simulink model "EM_SYS_simulink"  (R2021a)
settings: Solver=VariableStepAuto  StartTime=0.0  StopTime=10.0  MaxStep=0.001  RelTol=1e-3
values from neighbouring files (symbols this model uses):
  b = 0.2    [electro_mechanichal_model.m]
  J = 0.02    [electro_mechanichal_model.m]
  K = .015    (= 0.015)    [electro_mechanichal_model.m]
  Kb = .015    (= 0.015)    [electro_mechanichal_model.m]
  L = 0.5    [electro_mechanichal_model.m]
  R = 2.0    (= 2)    [electro_mechanichal_model.m]
settings Model: Creator=remon  LastModifiedBy=remon

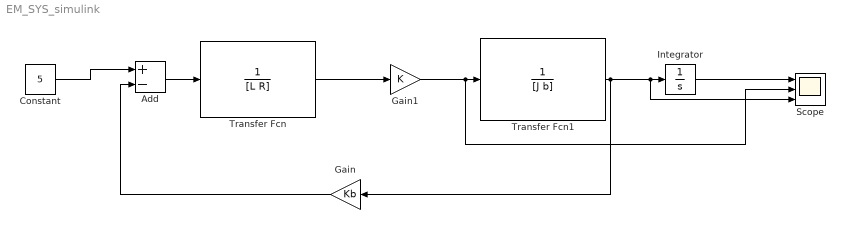
== system EM_SYS_simulink ==
  Add : Sum  Inputs=+-
  Constant : Constant  Value=5
  Gain : Gain  Gain=Kb
  Gain1 : Gain  Gain=K
  Integrator : Integrator
  Scope : Scope  NumInputPorts=3
  Transfer Fcn : TransferFcn  Denominator=[L R]
  Transfer Fcn1 : TransferFcn  Denominator=[J b]
  wires:
  Constant/1 -> Add/1
  Add/1 -> Transfer Fcn/1
  Transfer Fcn/1 -> Gain1/1
  Gain1/1 -> Scope/2, Transfer Fcn1/1
  Gain/1 -> Add/2
  Transfer Fcn1/1 -> Gain/1, Scope/3, Integrator/1
  Integrator/1 -> Scope/1
